simulink model "dlya_diploma_frontal"  (R2019b)
settings: Solver=VariableStepAuto  StartTime=0.0  StopTime=5  RelTol=1e-3
values from neighbouring files (symbols this model uses):
  A = [0 1 0 0; 68747/250 0 -29463/250 0; 0 0 0 1;-19642/125 0 9821/125 0]    [test_2.m]    (also in test_3.m = [0 1 0 0; 35856471/2703500 0 -2857911/1081400 0; 0 0 0 1;-98; test_4.m = subs(jacobian(x1, x),[te,te1,a,a1,OA,AB,mB,g],x_equi); test_5.m = [0 1 0 0; 9821/750 0 -9821/2250 0; 0 0 0 1;0 0 9821/375 0]; unicycle.m = [0 1 0 0; 0 0 0 0; 0 0 0 1;0 0 5588149/150160 0])
  B = [0; -16/15; 0; 16/15]    [test_2.m]    (also in test_3.m = [0; -2250/5407; 0; 6925/5407]; test_4.m = subs(jacobian(x1, sym('M')),[te,te1,a,a1,OA,AB,mB,g],x_equi); test_5.m = [0;  -8/15; 0; 8/5]; unicycle.m = [0;  6250/17; 0; -12500/1877])
  K = place(A,B,eigs)    [test_2.m]    (also in test_3.m; test_4.m; unicycle.m = acker(A,B,eigs); unicycle_fro.m = place(A,B,eigs1))
libraries: simulink x1
settings Model: Creator=DooDooDude  LastModifiedBy=DooDooDude

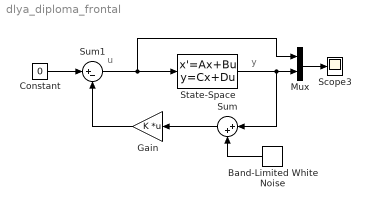
== system dlya_diploma_frontal ==
  note: u
  note: y
  Band-Limited White Noise : simulink/Sources/Band-Limited White Noise  Cov=[0 0 0 0]  Ts=0.005  seed=[23341]
  Constant : Constant  Value=0
  Gain : Gain  Gain=K  Multiplication=Matrix(K*u)
  Mux : Mux  Inputs=2
  Scope3 : Scope
  State-Space : StateSpace  A=A  B=B  C=eye(4)  D=[0; 0; 0; 0]  InitialCondition=[0; 0; 0.175; 0]
  Sum : Sum  Inputs=|++
  Sum1 : Sum  Inputs=|+-
  wires:
  State-Space/1 -> Sum/1, Mux/2
  Sum/1 -> Gain/1
  Band-Limited White Noise/1 -> Sum/2
  Gain/1 -> Sum1/2
  Sum1/1 -> Mux/1, State-Space/1
  Constant/1 -> Sum1/1
  Mux/1 -> Scope3/1
